simulink model "slexEntityTransportDelay_org"  (Simulink 10.0)
settings: Solver=VariableStepAuto  StartTime=0.0  StopTime=900  RelTol=1e-3
PostLoadFcn:
  | Simulink.defineIntEnumType('OperationMode', {'Idle', 'OnDemand', 'Max'}, [0; 1; 2]);
undefined symbols (not defined in the file): m, n
Description:
  | Modeling Cyber-Physical Systems
settings Model: Creator=The MathWorks, Inc.  LastModifiedBy=bhisma  EnablePacing=on  PacingRate=1000
settings DataIOCC: SaveFormat=Dataset  ReturnWorkspaceOutputs=on
settings OptimizationCC: LifeSpan=auto
settings DebuggingCC: UnderspecifiedInitializationDetection=Simplified  MergeDetectMultiDrivingBlocksExec=error  StrictBusMsg=ErrorOnBusTreatedAsVector  SymbolicDimsDataTypeCodeGenerationDiagnostic=none  SFUnexpectedBacktrackingDiag=error  SFNoUnconditionalDefaultTransitionDiag=error  SFExecutionAtInitializationDiag=warning  ArithmeticOperatorsInVariantConditions=error
settings HardwareCC: ProdBitPerPointer=64  ProdBitPerSizeT=64  ProdBitPerPtrDiffT=64  ProdLargestAtomicFloat=Float  ProdIntDivRoundTo=Zero  ProdEndianess=LittleEndian  ProdWordSize=64  ProdHWDeviceType=Intel->x86-64 (Windows64)
settings ModelReferenceCC: PropagateSignalLabelsOutOfModel=on
settings SFSimCC: SimUseLocalCustomCode=on  CustomCodeUndefinedFunction=FilterOut
settings RTWCC: RTWUseLocalCustomCode=on
settings CodeAppCC: StateflowObjectComments=off
settings GRTTargetCC: TargetLangStandard=C99 (ISO)  CombineOutputUpdateFcns=on  GRTInterface=off
settings ConfigComp: CovMetricSettings=dwe  CovHtmlReporting=off  CovSaveCumulativeToWorkspaceVar=off  CovSaveSingleToWorkspaceVar=off

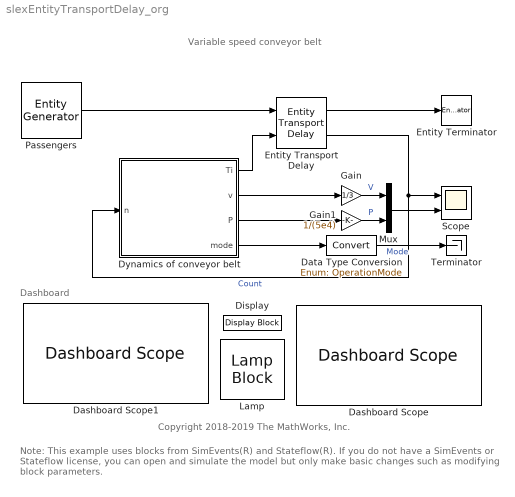
== system slexEntityTransportDelay_org ==
  note: Note: This example uses blocks from SimEvents(R) and Stateflow(R). If you do not have a SimEvents or Stateflow license, you can open and simulate the model but only make basic changes such as modifying block parameters.
  note: Dashboard
  note: Copyright 2018-2019 The MathWorks, Inc.
  note: Variable speed conveyor belt
  Dashboard Scope : DashboardScope  StatePerturbationForJacobian=auto  Ymin=0  Ymax=110
  Dashboard Scope1 : DashboardScope  StatePerturbationForJacobian=auto  Ymin=0  Ymax=1.1000000000000001
  Data Type Conversion : DataTypeConversion  StatePerturbationForJacobian=auto  OutDataTypeStr=Enum: OperationMode
  Display : DisplayBlock  StatePerturbationForJacobian=auto  LabelPosition=Hide  Format=short  Transparency=1
  Dynamics of conveyor belt : Stateflow chart  StatePerturbationForJacobian=auto  BlockKeywords=__PRM__SERIALIZED__DATA__:Stateflow Chart,Stateflow Diagram  TreatAsAtomicUnit=on
  Entity Transport Delay : EntityTransportDelay  StatePerturbationForJacobian=auto  InputPortMessageModes=m,n  OutputPortMessageModes=m,n  ShowNumberEntitiesInBlock=on
  Entity Terminator : EntityTerminator  StatePerturbationForJacobian=auto  InputPortMessageModes=m
  Gain : Gain  StatePerturbationForJacobian=auto  Gain=1/3
  Gain1 : Gain  StatePerturbationForJacobian=auto  Gain=1/(5e4)
  Lamp : LampBlock  StatePerturbationForJacobian=auto  DefaultColor=DataTag4  States=DataTag5
  Mux : Mux  StatePerturbationForJacobian=auto  Inputs=2
  Passengers : EntityGenerator  StatePerturbationForJacobian=auto  OutputPortMessageModes=m  TimeSource=MATLAB action  Period=0.1  IntergenerationTimeAction=|  GenerateEntityAtSimulationStart=off  EntityType=Structured  EntityTypeName=Entity
      | persistent rngInit;
      | if isempty(rngInit)
      |     seed = 12345;
      |     rng(seed);
      |     rngInit = true;
      | end
      | 
      | % Pattern: Exponential distribution
      | persistent time;
      | if isempty(time)
      |     time = 0;
      | end
      | if time < 180
      |     lambda = 2;
      | elseif time < 240
      |     lambda = .5;
      | elseif time < 300
      |     lambda = .1;
      | else
      |     time = 0;
      |     lambda = 2;
      | end
      | % Use inverse transform sampling to
      | % generate dt according to the exponential
      | % distribution
      | dt = -1/lambda * log(1 - rand());
      | time = time + dt;
      mask Display: image('$imagefile'); % Use "Edit Image" on toolstrip to change.
  Scope : Scope  NumInputPorts=2
      settings: StatePerturbationForJacobian=auto
  Terminator : Terminator
      settings: StatePerturbationForJacobian=auto
  wires:
  Entity Transport Delay/1 -> Entity Terminator/1
  Dynamics of conveyor belt/1(Ti) -> Entity Transport Delay/2
  Entity Transport Delay/2 -> Dynamics of conveyor belt/1(n), Scope/1  "Count"
  Dynamics of conveyor belt/2(v) -> Gain/1
  Dynamics of conveyor belt/3(P) -> Gain1/1
  Dynamics of conveyor belt/4(mode) -> Data Type Conversion/1
  Passengers/1 -> Entity Transport Delay/1
  Data Type Conversion/1 -> Terminator/1  "Mode"
  Gain/1 -> Mux/1  "V"
  Gain1/1 -> Mux/2  "P"
  Mux/1 -> Scope/2

== stateflow chart Dynamics of conveyor belt ==
  note: ?
  state Idle
    % no load
    Ti=100;
    v=1/Ti*L;
    P=(mu*n+fBelt)*v;
    mode=0;
  state OnDemand
    % keep speed
    Ti=L/V;
    v=V;
    P=(mu*n+fBelt)*v;
    mode=1;
  state Max
    % keep power
    v=maxPower/(mu*n+fBelt);
    Ti = L/v;
    P=(mu*n+fBelt)*v;
    mode=2;
  (default) -> Idle : {
      | % initialize local parameters
      | aveMass = 75;
      | mu = 0.5*10*aveMass; % *mu*g*aveMass, [N]
      | maxPower = 5e4; % maximum power, [W]
      | V = 3; % normal mode velocity, [m/s]
      | L = 50; % length of belt, [L]
      | fBelt = 1e4; % friction of zero load, [N]
      | }
  Idle -> OnDemand : [n*aveMass >= 10]
  OnDemand -> Max [order 2] : [(maxPower/V-fBelt)/mu  <= n]
  OnDemand -> Idle [order 1] : [n*aveMass < 10]
  Max -> OnDemand : [(maxPower/V-fBelt)/mu > n]
  data: Ti output double; n input double; mu local double =50; maxPower local double =5e4; V local double =3; L local double =50; fBelt local double =1e4; v output double; P output double; mode output int8; aveMass local double
